simulink model "demoAUVdepthPIDcontrol"  (R2023a)
settings: Solver=VariableStepAuto  StartTime=0.0  StopTime=400  RelTol=1e-3
libraries: slpidlib x1, mssSimulink x1
settings Model: Creator=23147  LastModifiedBy=23147

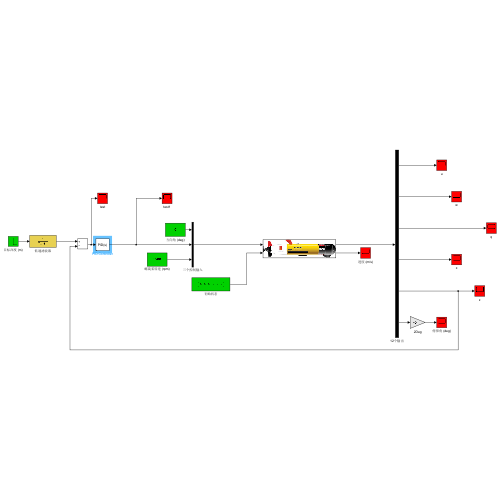
[thumbnail: Simulink's stored preview of the top-level diagram]
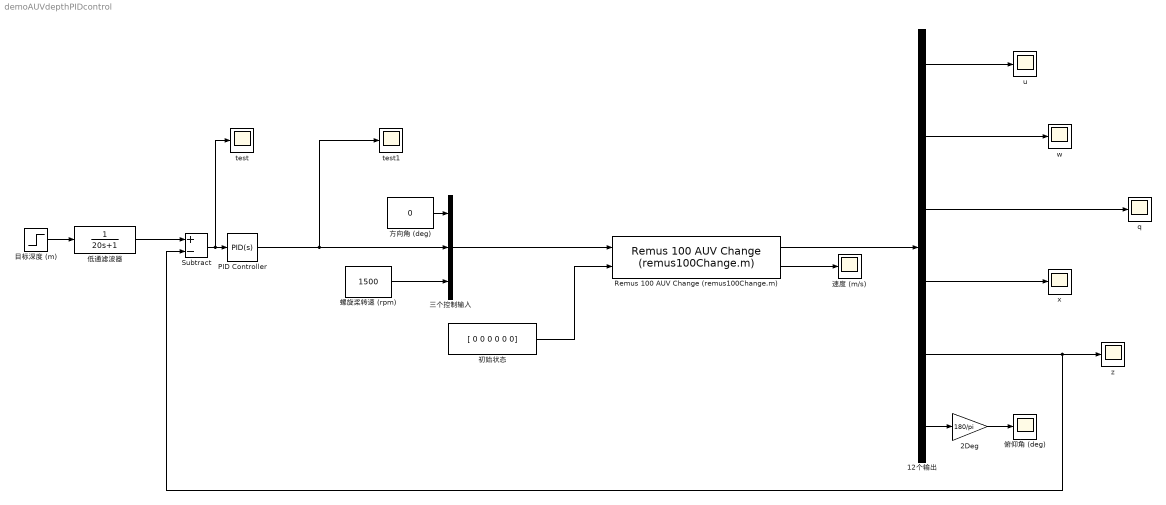
== system demoAUVdepthPIDcontrol ==
  12个输出 : Demux  Outputs=6
  2Deg : Gain  Gain=180/pi
  PID Controller : slpidlib/PID Controller  Controller=PID  Form=Parallel  TimeDomain=Continuous-time  UseExternalTs=off  SampleTime=-1  IntegratorMethod=Forward Euler  FilterMethod=Forward Euler  ControllerParametersSource=internal  P=-100  I=-0.01  UseKiTs=off  D=-500  N=100  UseFilter=on  TunerSelectOption=Transfer Function Based (PID Tuner App)  InitialConditionSource=internal  InitialConditionForIntegrator=0  InitialConditionForFilter=0  DifferentiatorICPrevScaledInput=0  ExternalReset=none  TrackingMode=off  Kt=1  LimitOutput=off  SatLimitsSource=internal  UpperSaturationLimit=inf  LowerSaturationLimit=-inf  LinearizeAsGain=on  AntiWindupMode=none  Kb=1  LimitIntegrator=off  UpperIntegratorSaturationLimit=inf  LowerIntegratorSaturationLimit=-inf  POutMin=[]  POutMax=[]  IOutMin=[]  IOutMax=[]  DOutMin=[]  DOutMax=[]  NOutMin=[]  NOutMax=[]  SumOutMin=[]  SumOutMax=[]  SaturationOutMin=[]  SaturationOutMax=[]  PParamMin=[]  PParamMax=[]  IParamMin=[]  IParamMax=[]  DParamMin=[]  DParamMax=[]  NParamMin=[]  NParamMax=[]  KbParamMin=[]  KbParamMax=[]  KtParamMin=[]  KtParamMax=[]  KbOutMin=[]  KbOutMax=[]  KtOutMin=[]  KtOutMax=[]  IntegratorOutMin=[]  IntegratorOutMax=[]  FilterOutMin=[]  FilterOutMax=[]  SumI1OutMin=[]  SumI1OutMax=[]  SumI2OutMin=[]  SumI2OutMax=[]  SumI3OutMin=[]  SumI3OutMax=[]  SumI4OutMin=[]  SumI4OutMax=[]  SumDOutMin=[]  SumDOutMax=[]  DifferentiatorOutMin=[]  DifferentiatorOutMax=[]  FilterDiffOutCoefMin=[]  FilterDiffOutCoefMax=[]  ReciprocalOutMin=[]  ReciprocalOutMax=[]  SumDenOutMin=[]  SumDenOutMax=[]  SumNumOutMin=[]  SumNumOutMax=[]  DivideOutMin=[]  DivideOutMax=[]  UdiffTsProdOutMin=[]  UdiffTsProdOutMax=[]  NTsProdOutMin=[]  NTsProdOutMax=[]  UintegralTsProdOutMin=[]  UintegralTsProdOutMax=[]  UngainTsProdOutMin=[]  UngainTsProdOutMax=[]  ClampingZeroOutDataTypeStr=Inherit: Inherit via back propagation  ClampingZeroOutMin=[]  ClampingZeroOutMax=[]  FilterDenConstantOutDataTypeStr=Inherit: Inherit via back propagation  FilterDenConstantOutMin=[]  FilterDenConstantOutMax=[]  PCopyOutDataTypeStr=Inherit: Inherit via back propagation  PCopyOutMin=[]  PCopyOutMax=[]  NCopyOutDataTypeStr=Inherit: Inherit via back propagation  NCopyOutMin=[]  NCopyOutMax=[]  IntegratorContinuousStateAttributes=''  IntegratorStateMustResolveToSignalObject=off  IntegratorRTWStateStorageClass=Auto  FilterContinuousStateAttributes=''  FilterStateMustResolveToSignalObject=off  FilterRTWStateStorageClass=Auto  ParallelPVariant=InternalParameters  IdealPVariant=Disabled  IVariant=InternalParameters  DVariant=InternalParameters  IntegratorVariant=Continuous  SatVariant=Disabled  AWVariant=Passthrough  PCopyVariant=Disabled  TRVariant=Disabled  FdbkBlocksVariant=Forward  IdealPFdbkVariant=Disabled  SatFdbkVariant=Disabled  DerivativeFilterVariant=ContFilter  NVariant=InternalParameters  NCopyVariant=Disabled  FilterICVariant=InternalICsFilter  IntegratorICVariant=InternalICs  ExternalResetVariant=Disabled  TRSumVariant=Passthrough  SumFdbkVariant=Disabled  SumVariant=Sum_PID  TsampFilterVariant=InternalTs  TsampNgainVariant=Passthrough  TsampIntegralVariant=Disabled_SignalSpec  ExternalSaturationOutDataTypeStr=Inherit: Same as second input
  Remus 100 AUV Change (remus100Change.m) : mssSimulink/Marine craft models/Remus 100 AUV Change (remus100Change.m)  SystemSampleTime=-1  VariantActivationTime=update diagram  Latency=0  AutoFrameSizeCalculation=off
  Subtract : Sum  Inputs=+-
  q : Scope
  test : Scope
  test1 : Scope
  u : Scope
  w : Scope
  x : Scope
  z : Scope
  三个控制输入 : Mux  Inputs=[1 1 1]
  低通滤波器 : TransferFcn  Denominator=[20 1]
  俯仰角 (deg) : Scope
  初始状态 : Constant  Value=[ 0 0 0 0 0 0]
  方向角 (deg) : Constant  Value=0
  目标深度 (m) : Step  Time=200  After=-30  SampleTime=0
  螺旋桨转速 (rpm) : Constant  Value=1500
  速度 (m/s) : Scope
  wires:
  初始状态/1 -> Remus 100 AUV Change (remus100Change.m)/2
  三个控制输入/1 -> Remus 100 AUV Change (remus100Change.m)/1
  螺旋桨转速 (rpm)/1 -> 三个控制输入/3
  方向角 (deg)/1 -> 三个控制输入/1
  目标深度 (m)/1 -> 低通滤波器/1
  Remus 100 AUV Change (remus100Change.m)/2 -> 速度 (m/s)/1
  Remus 100 AUV Change (remus100Change.m)/1 -> 12个输出/1
  12个输出/1 -> u/1
  12个输出/2 -> w/1
  12个输出/3 -> q/1
  12个输出/4 -> x/1
  12个输出/5 -> Subtract/2, z/1
  12个输出/6 -> 2Deg/1
  2Deg/1 -> 俯仰角 (deg)/1
  低通滤波器/1 -> Subtract/1
  Subtract/1 -> test/1, PID Controller/1
  PID Controller/1 -> test1/1, 三个控制输入/2
